simulink library "vehdynlibtirecommon"  (R2019b)
settings: Solver=ode45  StartTime=0.0  StopTime=10.0  RelTol=1e-3  EnableMultiTasking=on
undefined symbols (not defined in the file or in its folder): br, g, IYY, omegao, tireStruct, UNLOADED_RADIUS, VXLOW, zdoto, zo
libraries: autolibshared x3
Description:
  | Automotive Blockset Library: Components used in the Tire Dynamics Library
settings Model: ModifiedByFormat=The MathWorks, Inc.  Creator=The MathWorks, Inc.  LastModifiedBy=The MathWorks, Inc.
settings SolverCC: MinimalZcImpactIntegration=on
settings DataIOCC: LimitDataPoints=on  SaveFormat=Array  ReturnWorkspaceOutputs=off
settings OptimizationCC: LifeSpan=inf
settings DebuggingCC: AllowSymbolicDim=off  PregeneratedLibrarySubsystemCodeDiagnostic=none  SFUnexpectedBacktrackingDiag=warning  SFNoUnconditionalDefaultTransitionDiag=warning  SFExecutionAtInitializationDiag=none  ArithmeticOperatorsInVariantConditions=warning
settings HardwareCC: ProdBitPerPointer=32  ProdBitPerSizeT=32  ProdBitPerPtrDiffT=32  ProdLargestAtomicFloat=None  ProdIntDivRoundTo=Undefined  ProdEndianess=Unspecified  ProdWordSize=32  ProdHWDeviceType=32-bit Generic
settings ModelReferenceCC: PropagateSignalLabelsOutOfModel=off
settings SFSimCC: SimUseLocalCustomCode=off  CustomCodeUndefinedFunction=UseInterfaceOnly
settings RTWCC: RTWUseLocalCustomCode=off
settings CodeAppCC: StateflowObjectComments=on
settings GRTTargetCC: TargetLangStandard=C89/C90 (ANSI)  GeneratePreprocessorConditionals=Disable all
settings ConfigComp: CovMetricSettings=dw  CovHtmlReporting=on  CovSaveCumulativeToWorkspaceVar=on  CovSaveSingleToWorkspaceVar=on  CovShowResultsExplorer=off  CovExternalEMLEnable=off

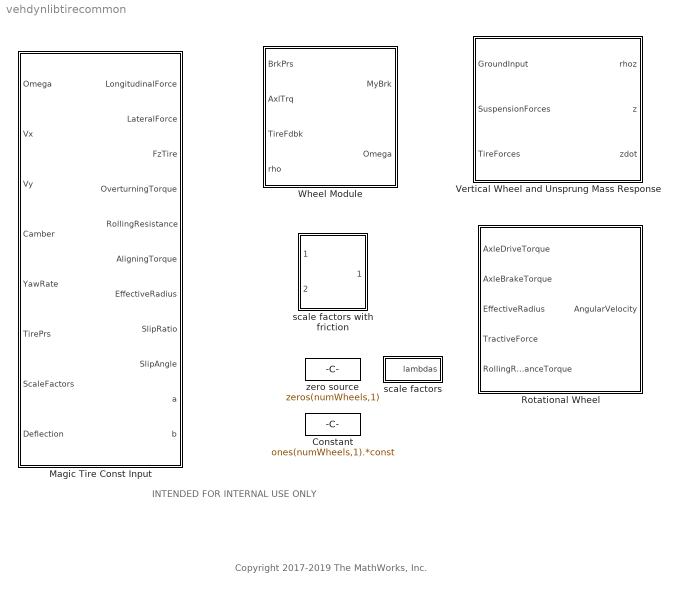
== system vehdynlibtirecommon ==
  note: INTENDED FOR INTERNAL USE ONLY
  note: Copyright 2017-2019 The MathWorks, Inc.
  Constant : Constant  Value=ones(numWheels,1).*const  mask{const=220000, numWheels=1}
      mask prompts: const "Constant Value"; numWheels "Number of wheels"
  Magic Tire Const Input : Subsystem
  Rotational Wheel : Subsystem  mask{Iyy=tireStruct(:).IYY, rhodot_o=omegao, br=br}
      mask prompts: Iyy "Wheel inertia [kg*m^2]"; rhodot_o "Initial wheel velocity [rad/s]"; br "Rotational damping [N*m*s/rad]"
  Vertical Wheel and Unsprung Mass Response : Subsystem  mask{m=tireStruct(:).MASS, bz=vertcat(tireStruct(:).VERTICAL_DAMPING), zo=zo, zdoto=zdoto, g=g, ReMax=.15}
      mask prompts: m "Unsprung mass [m]"; bz "Vertical damping [N*m/s]"; zo "Initial deflection [m]"; zdoto "Initial velocity [m/s]"; g "Gravitational acceleration [m/s^2]"; ReMax "Maximum unloaded radius [m]:"
  Wheel Module : Subsystem  mask{Iyy=IYY}
      mask prompts: Iyy "Rotational inertia, Iyy [kg*m^2]:"
  scale factors : Subsystem  mask{numWheels=1}
      mask prompts: numWheels "Number of wheels"
  scale factors with friction : Subsystem  mask{numWheels=1}
      mask prompts: numWheels "Number of wheels"
  zero source : Constant  Value=zeros(numWheels,1)  mask{numWheels=1}
      mask prompts: numWheels "Number of wheels"

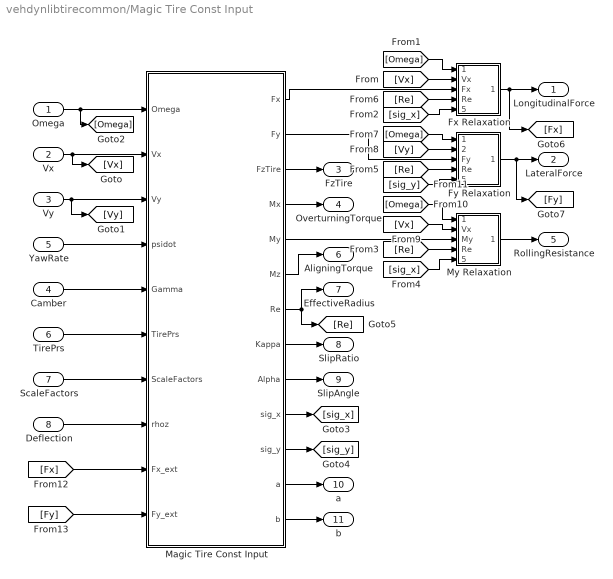
== system vehdynlibtirecommon/Magic Tire Const Input ==
  Omega : Inport
  Vx : Inport  Port=2
  Vy : Inport  Port=3
  Camber : Inport  Port=4
  YawRate : Inport  Port=5
  TirePrs : Inport  Port=6
  ScaleFactors : Inport  Port=7
  Deflection : Inport  Port=8
  Fx Relaxation : Subsystem
  Fy Relaxation : Subsystem
  Magic Tire Const Input : MATLAB Function
  My Relaxation : Subsystem  mask{UpperValue=VXLOW}
      mask prompts: UpperValue "Simulink:blkprm_prompts:DeadZoneEndOfDeadZone"
      mask TypeOptions UpperValue: Dead Zone/UpperValue
      mask DialogControl UpperValue Prompt: End of dead zone:
  LongitudinalForce : Outport  VectorParamsAs1DForOutWhenUnconnected=off
  LateralForce : Outport  Port=2  VectorParamsAs1DForOutWhenUnconnected=off
  FzTire : Outport  Port=3  VectorParamsAs1DForOutWhenUnconnected=off
  OverturningTorque : Outport  Port=4  VectorParamsAs1DForOutWhenUnconnected=off
  RollingResistance : Outport  Port=5  VectorParamsAs1DForOutWhenUnconnected=off
  AligningTorque : Outport  Port=6  VectorParamsAs1DForOutWhenUnconnected=off
  EffectiveRadius : Outport  Port=7  VectorParamsAs1DForOutWhenUnconnected=off
  SlipRatio : Outport  Port=8  VectorParamsAs1DForOutWhenUnconnected=off
  SlipAngle : Outport  Port=9  VectorParamsAs1DForOutWhenUnconnected=off
  a : Outport  Port=10  VectorParamsAs1DForOutWhenUnconnected=off
  b : Outport  Port=11  VectorParamsAs1DForOutWhenUnconnected=off
  wires:
  Magic Tire Const Input/3(FzTire) -> FzTire/1
  Omega/1 -> Magic Tire Const Input/1(Omega), [Omega]
  YawRate/1 -> Magic Tire Const Input/4(psidot)
  Camber/1 -> Magic Tire Const Input/5(Gamma)
  TirePrs/1 -> Magic Tire Const Input/6(TirePrs)
  ScaleFactors/1 -> Magic Tire Const Input/7(ScaleFactors)
  Deflection/1 -> Magic Tire Const Input/8(rhoz)
  Magic Tire Const Input/4(Mx) -> OverturningTorque/1
  Magic Tire Const Input/6(Mz) -> AligningTorque/1
  Magic Tire Const Input/8(Kappa) -> SlipRatio/1
  Magic Tire Const Input/9(Alpha) -> SlipAngle/1
  Magic Tire Const Input/2(Fy) -> Fy Relaxation/3(Fy)
  Magic Tire Const Input/7(Re) -> [Re], EffectiveRadius/1
  Fx Relaxation/1(Out1) -> LongitudinalForce/1, [Fx]
  My Relaxation/1(Out1) -> RollingResistance/1
  Vx/1 -> [Vx], Magic Tire Const Input/2(Vx)
  Vy/1 -> [Vy], Magic Tire Const Input/3(Vy)
  Magic Tire Const Input/5(My) -> My Relaxation/3(My)
  Magic Tire Const Input/13(b) -> b/1
  Magic Tire Const Input/12(a) -> a/1
  Fy Relaxation/1(Out1) -> [Fy], LateralForce/1
  [Vx] -> Fx Relaxation/2(Vx)
  [Omega] -> Fx Relaxation/1(omega)
  Magic Tire Const Input/10(sig_x) -> [sig_x]
  Magic Tire Const Input/11(sig_y) -> [sig_y]
  [sig_x] -> Fx Relaxation/5(sig_x)
  [Re] -> My Relaxation/4(Re)
  [sig_x] -> My Relaxation/5(sig_x)
  [Re] -> Fy Relaxation/4(Re)
  [Re] -> Fx Relaxation/4(Re)
  [Omega] -> Fy Relaxation/1(omega)
  [Vy] -> Fy Relaxation/2(Vsy)
  [Vx] -> My Relaxation/2(Vx)
  [Omega] -> My Relaxation/1(omega)
  [sig_y] -> Fy Relaxation/5(sig_y)
  Magic Tire Const Input/1(Fx) -> Fx Relaxation/3(Fx)
  [Fx] -> Magic Tire Const Input/9(Fx_ext)
  [Fy] -> Magic Tire Const Input/10(Fy_ext)

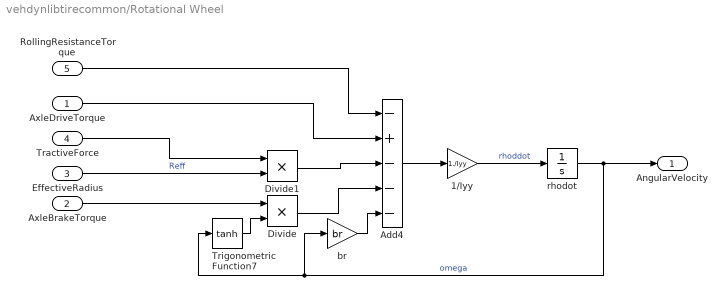
== system vehdynlibtirecommon/Rotational Wheel ==
  AxleDriveTorque : Inport
  AxleBrakeTorque : Inport  Port=2
  EffectiveRadius : Inport  Port=3
  TractiveForce : Inport  Port=4
  RollingResistanceTorque : Inport  Port=5
  1/Iyy : Gain  Gain=1./Iyy
  Add4 : Sum  Inputs=-+---
  Divide : Product  Inputs=**
  Divide1 : Product  Inputs=**
  Trigonometric Function7 : Trigonometry  Operator=tanh
  br : Gain  Gain=br
  "rhodot " : Integrator  InitialCondition=rhodot_o
  AngularVelocity : Outport  VectorParamsAs1DForOutWhenUnconnected=off
  wires:
  RollingResistanceTorque/1 -> Add4/1
  br/1 -> Add4/5
  AxleBrakeTorque/1 -> Divide/1
  AxleDriveTorque/1 -> Add4/2
  "rhodot "/1 -> AngularVelocity/1, Trigonometric Function7/1, br/1  "omega"
  Divide1/1 -> Add4/3
  EffectiveRadius/1 -> Divide1/2  "Reff"
  TractiveForce/1 -> Divide1/1
  Trigonometric Function7/1 -> Divide/2
  Divide/1 -> Add4/4
  Add4/1 -> 1/Iyy/1
  1/Iyy/1 -> "rhodot "/1  "rhoddot"

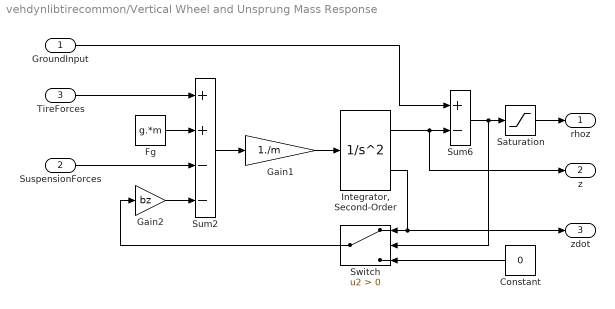
== system vehdynlibtirecommon/Vertical Wheel and Unsprung Mass Response ==
  GroundInput : Inport
  SuspensionForces : Inport  Port=2
  TireForces : Inport  Port=3
  Constant : Constant  Value=0
  Fg : Constant  Value=g.*m
  Gain1 : Gain  Gain=1./m  SaturateOnIntegerOverflow=on  OutDataTypeStr=Inherit: Same as input  ParamDataTypeStr=Inherit: Same as input
  Gain2 : Gain  Gain=bz  SaturateOnIntegerOverflow=on  OutDataTypeStr=Inherit: Same as input  ParamDataTypeStr=Inherit: Same as input
  "Integrator, Second-Order" : SecondOrderIntegrator  ICX=-zo  UpperLimitX=ReMax  LowerLimitX=0  ICDXDT=zdoto
  Saturation : Saturate  UpperLimit=inf  LowerLimit=0  ZeroCross=off
  Sum2 : Sum  Inputs=++--  SaturateOnIntegerOverflow=on  InputSameDT=on  OutDataTypeStr=Inherit: Same as first input
  Sum6 : Sum  Inputs=+-  SaturateOnIntegerOverflow=on  InputSameDT=on  OutDataTypeStr=Inherit: Same as first input
  Switch : Switch  Criteria=u2 > Threshold  ZeroCross=off
  rhoz : Outport  VectorParamsAs1DForOutWhenUnconnected=off
  z : Outport  Port=2  VectorParamsAs1DForOutWhenUnconnected=off
  zdot : Outport  Port=3  VectorParamsAs1DForOutWhenUnconnected=off
  wires:
  "Integrator, Second-Order"/2 -> zdot/1, Switch/1
  Gain2/1 -> Sum2/4
  Fg/1 -> Sum2/2
  Saturation/1 -> rhoz/1
  GroundInput/1 -> Sum6/1
  "Integrator, Second-Order"/1 -> Sum6/2, z/1
  Gain1/1 -> "Integrator, Second-Order"/1
  Sum2/1 -> Gain1/1
  SuspensionForces/1 -> Sum2/3
  TireForces/1 -> Sum2/1
  Sum6/1 -> Switch/2, Saturation/1
  Switch/1 -> Gain2/1
  Constant/1 -> Switch/3

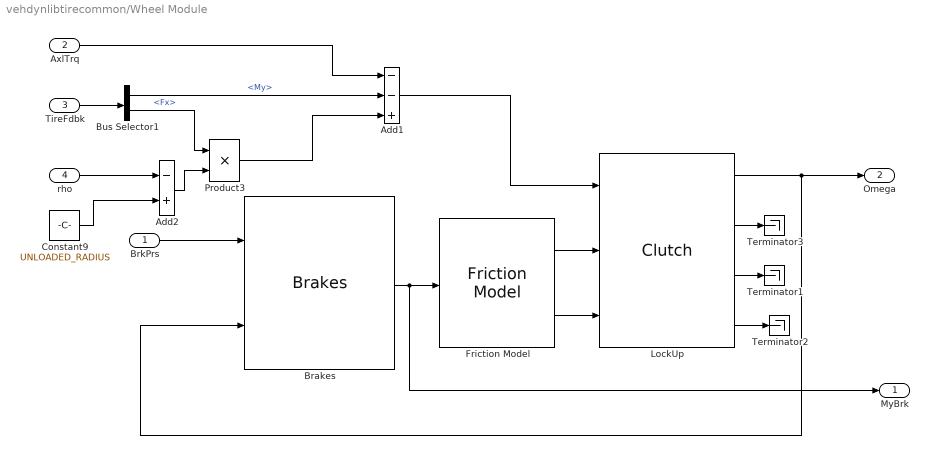
== system vehdynlibtirecommon/Wheel Module ==
  BrkPrs : Inport
  AxlTrq : Inport  Port=2
  TireFdbk : Inport  Port=3
  rho : Inport  Port=4
  Add1 : Sum  Inputs=--+
  Add2 : Sum  Inputs=-+
  Brakes : autolibshared/Longitudinal Wheel/Wheel Module/Brakes  SystemSampleTime=-1  LabelModeActiveChoice=Disk  Latency=0  AutoFrameSizeCalculation=off
      settings: SourceProductName=Powertrain Blockset  SourceProductBaseCode=PW
  Bus Selector1 : BusSelector  OutputSignals=My,Fx
  Constant9 : Constant  Value=UNLOADED_RADIUS
  Friction Model : autolibshared/Longitudinal Wheel/Wheel Module/Friction Model  SystemSampleTime=-1  Latency=0  AutoFrameSizeCalculation=off
      settings: SourceProductName=Powertrain Blockset  SourceProductBaseCode=PW
  LockUp : autolibshared/Longitudinal Wheel/Wheel Module/Clutch  OmegaTol=pi/30
      settings: SourceProductName=Powertrain Blockset  SourceProductBaseCode=PW
  Product3 : Product  Inputs=**
  Terminator1 : Terminator
  Terminator2 : Terminator
  Terminator3 : Terminator
  MyBrk : Outport  VectorParamsAs1DForOutWhenUnconnected=off
  Omega : Outport  Port=2  VectorParamsAs1DForOutWhenUnconnected=off
  wires:
  TireFdbk/1 -> Bus Selector1/1
  Bus Selector1/1 -> Add1/2  "<My>"
  Bus Selector1/2 -> Product3/1  "<Fx>"
  BrkPrs/1 -> Brakes/1
  AxlTrq/1 -> Add1/1
  rho/1 -> Add2/1
  Constant9/1 -> Add2/2
  Add2/1 -> Product3/2
  Product3/1 -> Add1/3
  LockUp/4 -> Terminator2/1
  Brakes/1 -> MyBrk/1, Friction Model/1
  Friction Model/2 -> LockUp/3
  LockUp/3 -> Terminator1/1
  LockUp/2 -> Terminator3/1
  Add1/1 -> LockUp/1
  LockUp/1 -> Omega/1, Brakes/2
  Friction Model/1 -> LockUp/2

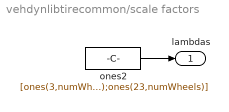
== system vehdynlibtirecommon/scale factors ==
  ones2 : Constant  Value=[ones(3,numWheels);zeros(1,numWheels);ones(23,numWheels)]
  lambdas : Outport  VectorParamsAs1DForOutWhenUnconnected=off
  wires:
  ones2/1 -> lambdas/1

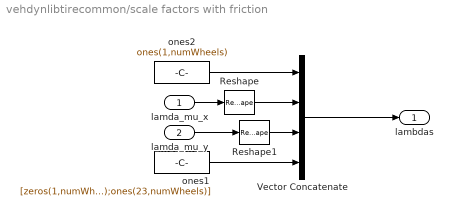
== system vehdynlibtirecommon/scale factors with friction ==
  lamda_mu_x : Inport
  lamda_mu_y : Inport  Port=2
  Reshape : Reshape  OutputDimensionality=Row vector (2-D)  OutputDimensions=[1,numWheels]
  Reshape1 : Reshape  OutputDimensionality=Row vector (2-D)  OutputDimensions=[1,numWheels]
  Vector Concatenate : Concatenate  NumInputs=4  Mode=Multidimensional array
  ones1 : Constant  Value=[zeros(1,numWheels);ones(23,numWheels)]  VectorParams1D=off
  ones2 : Constant  Value=ones(1,numWheels)  VectorParams1D=off
  lambdas : Outport  VectorParamsAs1DForOutWhenUnconnected=off
  wires:
  Reshape1/1 -> Vector Concatenate/3
  Reshape/1 -> Vector Concatenate/2
  lamda_mu_y/1 -> Reshape1/1
  lamda_mu_x/1 -> Reshape/1
  ones1/1 -> Vector Concatenate/4
  Vector Concatenate/1 -> lambdas/1
  ones2/1 -> Vector Concatenate/1

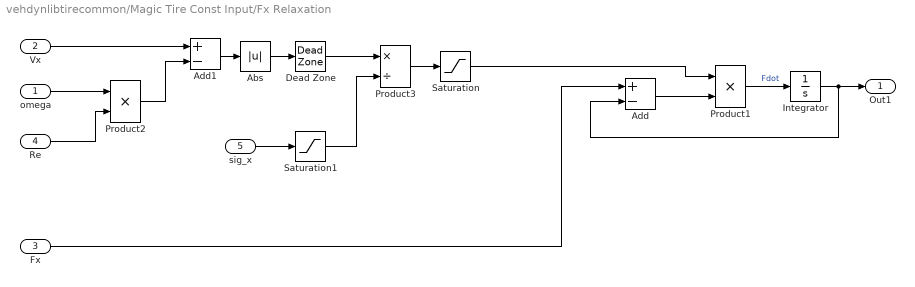
== system vehdynlibtirecommon/Magic Tire Const Input/Fx Relaxation ==
  omega : Inport
  Vx : Inport  Port=2
  Fx : Inport  Port=3
  Re : Inport  Port=4
  sig_x : Inport  Port=5
  Abs : Abs  ZeroCross=off
  Add : Sum  Inputs=+-
  Add1 : Sum  Inputs=+-
  Dead Zone : DeadZone  LowerValue=0  UpperValue=VXLOW  ZeroCross=off  SaturateOnIntegerOverflow=on
  Integrator : Integrator  UpperSaturationLimit=10e3  LowerSaturationLimit=-10e3  ZeroCross=off
  Product1 : Product  Inputs=**
  Product2 : Product  Inputs=**
  Product3 : Product  Inputs=*/
  Saturation : Saturate  UpperLimit=400*pi*2  LowerLimit=2*pi  ZeroCross=off
  Saturation1 : Saturate  UpperLimit=10  LowerLimit=.01  ZeroCross=off
  Out1 : Outport  PortDimensions=1  VectorParamsAs1DForOutWhenUnconnected=off
  wires:
  Abs/1 -> Dead Zone/1
  Product2/1 -> Add1/2
  Vx/1 -> Add1/1
  Product3/1 -> Saturation/1
  Re/1 -> Product2/2
  omega/1 -> Product2/1
  Fx/1 -> Add/1
  Integrator/1 -> Add/2, Out1/1
  Product1/1 -> Integrator/1  "Fdot"
  Add/1 -> Product1/2
  Add1/1 -> Abs/1
  Saturation/1 -> Product1/1
  Dead Zone/1 -> Product3/1
  sig_x/1 -> Saturation1/1
  Saturation1/1 -> Product3/2

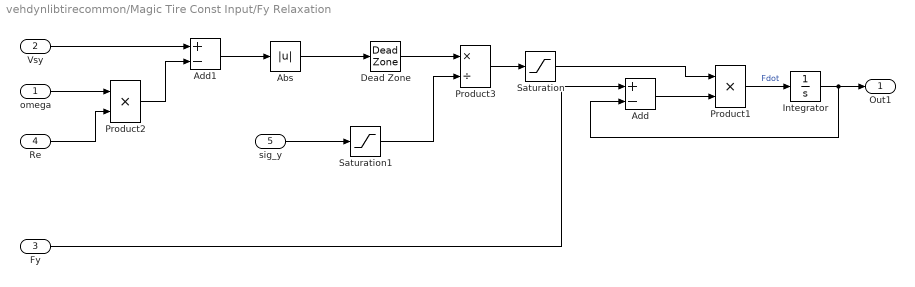
== system vehdynlibtirecommon/Magic Tire Const Input/Fy Relaxation ==
  omega : Inport
  Vsy : Inport  Port=2
  Fy : Inport  Port=3
  Re : Inport  Port=4
  sig_y : Inport  Port=5
  Abs : Abs  ZeroCross=off
  Add : Sum  Inputs=+-
  Add1 : Sum  Inputs=+-
  Dead Zone : DeadZone  LowerValue=0  UpperValue=VXLOW  ZeroCross=off  SaturateOnIntegerOverflow=on
  Integrator : Integrator  UpperSaturationLimit=10e3  LowerSaturationLimit=-10e3  AbsoluteTolerance=1e-3  ZeroCross=off
  Product1 : Product  Inputs=**
  Product2 : Product  Inputs=**
  Product3 : Product  Inputs=*/
  Saturation : Saturate  UpperLimit=400*pi  LowerLimit=2*pi  ZeroCross=off
  Saturation1 : Saturate  UpperLimit=10  LowerLimit=.01  ZeroCross=off
  Out1 : Outport  PortDimensions=1  VectorParamsAs1DForOutWhenUnconnected=off
  wires:
  Add/1 -> Product1/2
  Product1/1 -> Integrator/1  "Fdot"
  Integrator/1 -> Out1/1, Add/2
  Fy/1 -> Add/1
  omega/1 -> Product2/1
  Re/1 -> Product2/2
  Product3/1 -> Saturation/1
  Vsy/1 -> Add1/1
  Product2/1 -> Add1/2
  Saturation/1 -> Product1/1
  Abs/1 -> Dead Zone/1
  Dead Zone/1 -> Product3/1
  Add1/1 -> Abs/1
  sig_y/1 -> Saturation1/1
  Saturation1/1 -> Product3/2

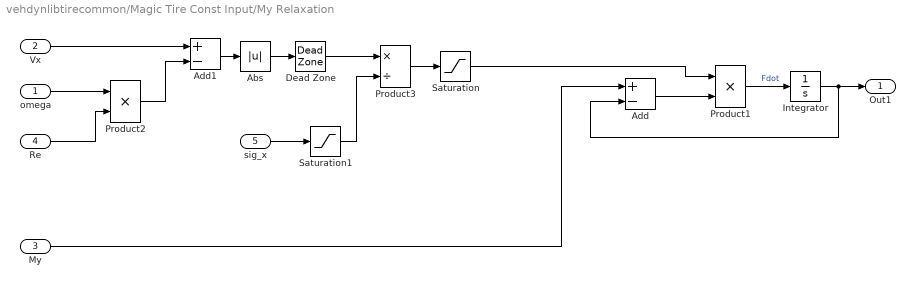
== system vehdynlibtirecommon/Magic Tire Const Input/My Relaxation ==
  omega : Inport
  Vx : Inport  Port=2
  My : Inport  Port=3
  Re : Inport  Port=4
  sig_x : Inport  Port=5
  Abs : Abs  ZeroCross=off
  Add : Sum  Inputs=+-
  Add1 : Sum  Inputs=+-
  Dead Zone : DeadZone  LowerValue=0  UpperValue=UpperValue  ZeroCross=off  SaturateOnIntegerOverflow=on
  Integrator : Integrator  UpperSaturationLimit=10e3  LowerSaturationLimit=-10e3  AbsoluteTolerance=1e-3  ZeroCross=off
  Product1 : Product  Inputs=**
  Product2 : Product  Inputs=**
  Product3 : Product  Inputs=*/
  Saturation : Saturate  UpperLimit=400*pi*2  LowerLimit=2*pi  ZeroCross=off
  Saturation1 : Saturate  UpperLimit=10  LowerLimit=.01  ZeroCross=off
  Out1 : Outport  PortDimensions=1  VectorParamsAs1DForOutWhenUnconnected=off
  wires:
  Dead Zone/1 -> Product3/1
  Saturation/1 -> Product1/1
  Add1/1 -> Abs/1
  Add/1 -> Product1/2
  Product1/1 -> Integrator/1  "Fdot"
  Integrator/1 -> Out1/1, Add/2
  My/1 -> Add/1
  omega/1 -> Product2/1
  Re/1 -> Product2/2
  Product3/1 -> Saturation/1
  Vx/1 -> Add1/1
  Product2/1 -> Add1/2
  Abs/1 -> Dead Zone/1
  sig_x/1 -> Saturation1/1
  Saturation1/1 -> Product3/2

== matlab function vehdynlibtirecommon/Magic Tire Const Input/Magic Tire Const Input ==
  data: Omega input; Vx input; Vy input; psidot input; Gamma input; TirePrs input; ScaleFactors input size=[27,1]; rhoz input; plySteer parameter; Fx output size=size(Omega); Fy output double size=size(Omega); FzTire output size=size(Omega); Mx output size=size(Omega); My output size=size(Omega); Mz output size=size(Omega); Re output size=size(Omega); Kappa output size=size(Omega); Alpha output size=size(Omega); sig_x output; sig_y output; PRESMAX parameter; PRESMIN parameter; FZMAX parameter; FZMIN parameter; VXLOW parameter; KPUMAX parameter; KPUMIN parameter; ALPMAX parameter; ALPMIN parameter; CAMMIN parameter; CAMMAX parameter; LONGVL parameter; UNLOADED_RADIUS parameter; NOMPRES parameter; FNOMIN parameter; VERTICAL_STIFFNESS parameter; DREFF parameter; BREFF parameter; FREFF parameter; Q_RE0 parameter; Q_V1 parameter; Q_V2 parameter; Q_FZ1 parameter; Q_FZ2 parameter; Q_FCX parameter; Q_FCY parameter; PFZ1 parameter; Q_FCY2 parameter; PCX1 parameter; PDX1 parameter; PDX2 parameter; PDX3 parameter; PEX1 parameter; PEX2 parameter; PEX3 parameter; PEX4 parameter; PKX1 parameter; PKX2 parameter; PKX3 parameter; PHX1 parameter; PHX2 parameter; PVX1 parameter; PVX2 parameter; PPX1 parameter; PPX2 parameter; PPX3 parameter; PPX4 parameter; RBX1 parameter; RBX2 parameter; RBX3 parameter; RCX1 parameter; REX1 parameter; REX2 parameter; RHX1 parameter; QSX1 parameter; QSX2 parameter; QSX3 parameter; QSX4 parameter; QSX5 parameter; QSX6 parameter; QSX7 parameter; QSX8 parameter; QSX9 parameter; QSX10 parameter; QSX11 parameter; PPMX1 parameter; PCY1 parameter; PDY1 parameter; PDY2 parameter; PDY3 parameter; PEY1 parameter; PEY2 parameter; PEY3 parameter; PEY4 parameter; PEY5 parameter; PKY1 parameter; PKY2 parameter; PKY3 parameter; PKY4 parameter; PKY5 parameter; PKY6 parameter; PKY7 parameter; PHY1 parameter; PHY2 parameter; PVY1 parameter; PVY2 parameter; PVY3 parameter; PVY4 parameter; PPY1 parameter; PPY2 parameter; PPY3 parameter; PPY4 parameter; PPY5 parameter; RBY1 parameter; RBY2 parameter; RBY3 parameter; RBY4 parameter; RCY1 parameter; REY1 parameter; REY2 parameter; RHY1 parameter; RHY2 parameter; RVY1 parameter; RVY2 parameter; RVY3 parameter; RVY4 parameter; RVY5 parameter; RVY6 parameter; QSY1 parameter; QSY2 parameter; QSY3 parameter; QSY4 parameter; QSY5 parameter; QSY6 parameter; QSY7 parameter; QSY8 parameter; QBZ1 parameter; QBZ2 parameter; QBZ3 parameter; QBZ4 parameter; QBZ5 parameter; QBZ6 parameter; QBZ9 parameter; QBZ10 parameter; QCZ1 parameter; QDZ1 parameter; QDZ2 parameter; QDZ3 parameter; QDZ4 parameter; QDZ6 parameter; QDZ7 parameter; QDZ8 parameter; QDZ9 parameter; QDZ10 parameter; QDZ11 parameter; QEZ1 parameter; QEZ2 parameter; QEZ3 parameter; QEZ4 parameter; QEZ5 parameter; QHZ1 parameter; QHZ2 parameter; QHZ3 parameter; QHZ4 parameter; PPZ1 parameter; PPZ2 parameter; SSZ1 parameter; SSZ2 parameter; SSZ3 parameter; SSZ4 parameter; PDXP1 parameter; PDXP2 parameter; PDXP3 parameter; PKYP1 parameter; PDYP1 parameter; PDYP2 parameter; PDYP3 parameter; PDYP4 parameter; PHYP1 parameter; PHYP2 parameter; PHYP3 parameter; PHYP4 parameter; PECP1 parameter; PECP2 parameter; QDTP1 parameter; QCRP1 parameter; QCRP2 parameter; QBRP1 parameter; QDRP1 parameter; QDRP2 parameter; WIDTH parameter; Q_RA1 parameter; Q_RA2 parameter; Q_RB1 parameter; Q_RB2 parameter; QSX12 parameter; QSX13 parameter; QSX14 parameter; a output; b output; Q_FZ3 parameter; LONGITUDINAL_STIFFNESS parameter; LATERAL_STIFFNESS parameter; PCFX1 parameter; PCFX2 parameter; PCFX3 parameter; PCFY1 parameter; PCFY2 parameter; PCFY3 parameter; Fx_ext input; Fy_ext input
function [Fx,Fy,FzTire,Mx,My,Mz,Re,Kappa,Alpha,sig_x,sig_y,a,b] = magictire(Omega,Vx,Vy,psidot,Gamma,TirePrs,ScaleFactors,rhoz,plySteer,...
PRESMAX,...
PRESMIN,...
FZMAX,...
FZMIN,...
VXLOW,...
KPUMAX,...
KPUMIN,...
ALPMAX,...
ALPMIN,...
CAMMIN,...
CAMMAX,...
LONGVL,...
UNLOADED_RADIUS,...
NOMPRES,...
FNOMIN,...
VERTICAL_STIFFNESS,...% vertical
DREFF,...
BREFF,...
FREFF,...
Q_RE0,...
Q_V1,...
Q_V2,...
Q_FZ1,...
Q_FZ2,...
Q_FCX,...
Q_FCY,...
PFZ1,...
Q_FCY2,...
PCX1,...% longitudinal
PDX1,...
PDX2,...
PDX3,...
PEX1,...
PEX2,...
PEX3,...
PEX4,...
PKX1,...
PKX2,...
PKX3,...
PHX1,...
PHX2,...
PVX1,...
PVX2,...
PPX1,...
PPX2,...
PPX3,...
PPX4,...
RBX1,...
RBX2,...
RBX3,...
RCX1,...
REX1,...
REX2,...
RHX1,...
QSX1,...% overturning
QSX2,...
QSX3,...
QSX4,...
QSX5,...
QSX6,...
QSX7,...
QSX8,...
QSX9,...
QSX10,...
QSX11,...
PPMX1,...
PCY1,...% lateral
PDY1,...
PDY2,...
PDY3,...
PEY1,...
PEY2,...
PEY3,...
PEY4,...
PEY5,...
PKY1,...
PKY2,...
PKY3,...
PKY4,...
PKY5,...
PKY6,...
PKY7,...
PHY1,...
PHY2,...
PVY1,...
PVY2,...
PVY3,...
PVY4,...
PPY1,...
PPY2,...
PPY3,...
PPY4,...
PPY5,...
RBY1,...
RBY2,...
RBY3,...
RBY4,...
RCY1,...
REY1,...
REY2,...
RHY1,...
RHY2,...
RVY1,...
RVY2,...
RVY3,...
RVY4,...
RVY5,...
RVY6,...
QSY1,...% rolling
QSY2,...
QSY3,...
QSY4,...
QSY5,...
QSY6,...
QSY7,...
QSY8,...
QBZ1,...
QBZ2,...
QBZ3,...
QBZ4,...
QBZ5,...
QBZ6,...
QBZ9,...
QBZ10,...
QCZ1,...
QDZ1,...
QDZ2,...
QDZ3,...
QDZ4,...
QDZ6,...
QDZ7,...
QDZ8,...
QDZ9,...
QDZ10,...
QDZ11,...
QEZ1,...
QEZ2,...
QEZ3,...
QEZ4,...
QEZ5,...
QHZ1,...
QHZ2,...
QHZ3,...
QHZ4,...
PPZ1,...
PPZ2,...
SSZ1,...
SSZ2,...
SSZ3,...
SSZ4,...
PDXP1,...% turn slip
PDXP2,...
PDXP3,...
PKYP1,...
PDYP1,...
PDYP2,...
PDYP3,...
PDYP4,...
PHYP1,...
PHYP2,...
PHYP3,...
PHYP4,...
PECP1,...
PECP2,...
QDTP1,...
QCRP1,...% aligning moment
QCRP2,...
QBRP1,...
QDRP1,...
QDRP2,...
WIDTH,...
Q_RA1,... % contact patch
Q_RA2,...
Q_RB1,...
Q_RB2,...
QSX12,...
QSX13,...
QSX14,...
Q_FZ3,...
LONGITUDINAL_STIFFNESS,...% structural
LATERAL_STIFFNESS,...
PCFX1,...
PCFX2,...
PCFX3,...
PCFY1,...
PCFY2,...
PCFY3,...
Fx_ext,...
Fy_ext)
%#codegen
coder.allowpcode('plain')
[Fx,Fy,FzTire,Mx,My,Mz,Re,Kappa,Alpha,sig_x,sig_y,a,b] = vdyncsmtire(Omega,Vx,Vy,psidot,Gamma,TirePrs,ScaleFactors,rhoz,plySteer,...
PRESMAX,...
PRESMIN,...
FZMAX,...
FZMIN,...
VXLOW,...
KPUMAX,...
KPUMIN,...
ALPMAX,...
ALPMIN,...
CAMMIN,...
CAMMAX,...
LONGVL,...
UNLOADED_RADIUS,...
NOMPRES,...
FNOMIN,...
VERTICAL_STIFFNESS,...% vertical
DREFF,...
BREFF,...
FREFF,...
Q_RE0,...
Q_V1,...
Q_V2,...
Q_FZ1,...
Q_FZ2,...
Q_FCX,...
Q_FCY,...
PFZ1,...
Q_FCY2,...
PCX1,...% longitudinal
PDX1,...
PDX2,...
PDX3,...
PEX1,...
PEX2,...
PEX3,...
PEX4,...
PKX1,...
PKX2,...
PKX3,...
PHX1,...
PHX2,...
PVX1,...
PVX2,...
PPX1,...
PPX2,...
PPX3,...
PPX4,...
RBX1,...
RBX2,...
RBX3,...
RCX1,...
REX1,...
REX2,...
RHX1,...
QSX1,...% overturning
QSX2,...
QSX3,...
QSX4,...
QSX5,...
QSX6,...
QSX7,...
QSX8,...
QSX9,...
QSX10,...
QSX11,...
PPMX1,...
PCY1,...% lateral
PDY1,...
PDY2,...
PDY3,...
PEY1,...
PEY2,...
PEY3,...
PEY4,...
PEY5,...
PKY1,...
PKY2,...
PKY3,...
PKY4,...
PKY5,...
PKY6,...
PKY7,...
PHY1,...
PHY2,...
PVY1,...
PVY2,...
PVY3,...
PVY4,...
PPY1,...
PPY2,...
PPY3,...
PPY4,...
PPY5,...
RBY1,...
RBY2,...
RBY3,...
RBY4,...
RCY1,...
REY1,...
REY2,...
RHY1,...
RHY2,...
RVY1,...
RVY2,...
RVY3,...
RVY4,...
RVY5,...
RVY6,...
QSY1,...% rolling
QSY2,...
QSY3,...
QSY4,...
QSY5,...
QSY6,...
QSY7,...
QSY8,...
QBZ1,...
QBZ2,...
QBZ3,...
QBZ4,...
QBZ5,...
QBZ6,...
QBZ9,...
QBZ10,...
QCZ1,...
QDZ1,...
QDZ2,...
QDZ3,...
QDZ4,...
QDZ6,...
QDZ7,...
QDZ8,...
QDZ9,...
QDZ10,...
QDZ11,...
QEZ1,...
QEZ2,...
QEZ3,...
QEZ4,...
QEZ5,...
QHZ1,...
QHZ2,...
QHZ3,...
QHZ4,...
PPZ1,...
PPZ2,...
SSZ1,...
SSZ2,...
SSZ3,...
SSZ4,...
PDXP1,...% turn slip
PDXP2,...
PDXP3,...
PKYP1,...
PDYP1,...
PDYP2,...
PDYP3,...
PDYP4,...
PHYP1,...
PHYP2,...
PHYP3,...
PHYP4,...
PECP1,...
PECP2,...
QDTP1,...
QCRP1,...% aligning moment
QCRP2,...
QBRP1,...
QDRP1,...
QDRP2,...
WIDTH,...
Q_RA1,... % contact patch
Q_RA2,...
Q_RB1,...
Q_RB2,...
QSX12,...
QSX13,...
QSX14,...
Q_FZ3,...
LONGITUDINAL_STIFFNESS,...% structural
LATERAL_STIFFNESS,...
PCFX1,...
PCFX2,...
PCFX3,...
PCFY1,...
PCFY2,...
PCFY3,...
Fx_ext,...
Fy_ext);
end
